simulink model "LUPA_Array_Eqk_circuit_w_PTO_DC_link_v2"  (R2024b)
settings: Solver=VariableStepAuto  StartTime=0.0  StopTime=20  RelTol=1e-5
values from neighbouring files (symbols this model uses):
  B = permute(B,  [3 2 1])    [convh5_v2.m]
  Hs = app.HsField.Value    [WEC_Sankey_App.m]    (also in build_sankey_postprocess.m = output.Hs.x)
  rx = app.DampingField.Value    [WEC_Sankey_App.m]
  sc_factor = 20    [Loss_analysis.m]
  Tp = app.TeField.Value    [WEC_Sankey_App.m]
undefined symbols (not defined in the file or in its folder): C_f1, C_f2, Fex_f1, Fex_f2, hydro, L_hs_f2, lambda, pp, R_cable, R_cable_scaled, R_rad_f1, R_rad_f2, Rs
libraries: fl_lib x41, nesl_utility x24, ee_lib x9
settings Model: Creator=inyongkim  LastModifiedBy=inyongkim
settings DebuggingCC: AlgebraicLoopMsg=none

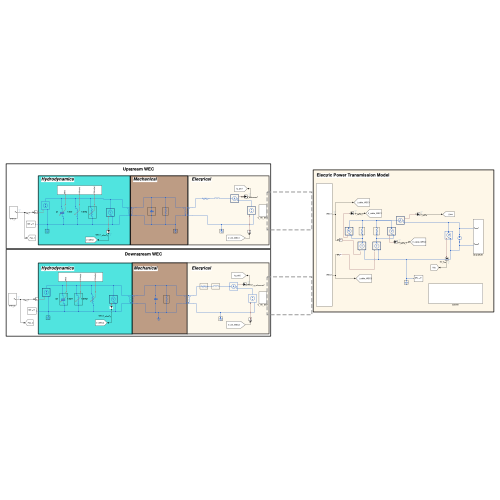
[thumbnail: Simulink's stored preview of the top-level diagram]
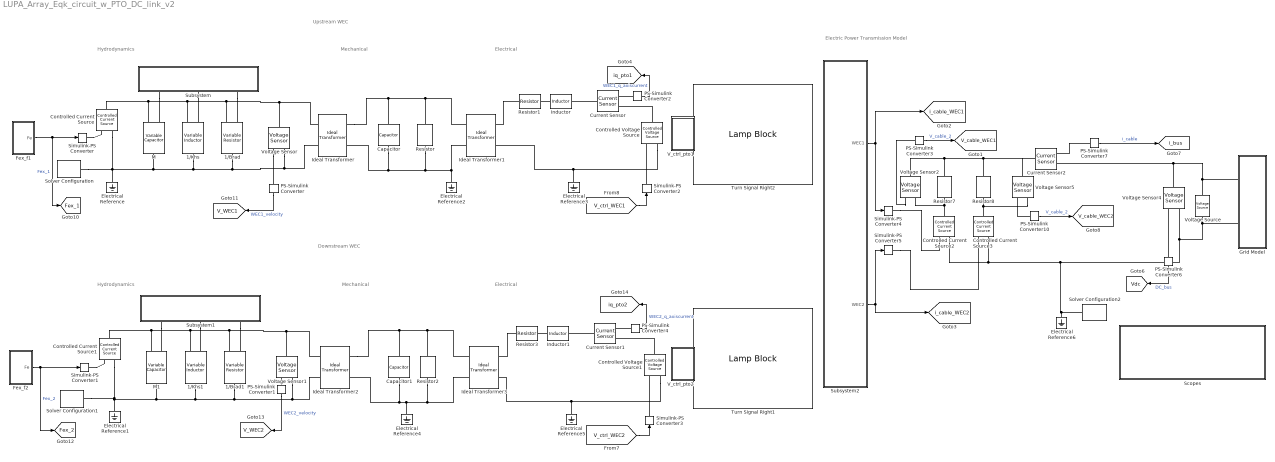
== system LUPA_Array_Eqk_circuit_w_PTO_DC_link_v2 ==
  note: Electrical
  note: Mechanical
  note: Hydrodynamics
  note: Electrical
  note: Mechanical
  note: Hydrodynamics
  note: Electric Power Transmission Model
  note: Upstream WEC
  note: Downstream WEC
  1/Brad : fl_lib/Electrical/Electrical Elements/Variable Resistor  Rmin=0 Ohm  thermalEnable=false  thermal_mass=1 J/K  i_specify=off  i_priority=None  i=0 A  i_nominal_specify=off  i_nominal_value=1  i_nominal_unit=A  v_specify=off  v_priority=None  v=0 V  v_nominal_specify=off  v_nominal_value=1  v_nominal_unit=V  T_specify=off  T_priority=None  T=300 K  T_nominal_specify=off  T_nominal_value=1  T_nominal_unit=K
  1/Brad1 : fl_lib/Electrical/Electrical Elements/Variable Resistor  Rmin=0 Ohm  thermalEnable=false  thermal_mass=1 J/K  i_specify=off  i_priority=None  i=0 A  i_nominal_specify=off  i_nominal_value=1  i_nominal_unit=A  v_specify=off  v_priority=None  v=0 V  v_nominal_specify=off  v_nominal_value=1  v_nominal_unit=V  T_specify=off  T_priority=None  T=300 K  T_nominal_specify=off  T_nominal_value=1  T_nominal_unit=K
  1/Khs : ee_lib/Passive/Variable Inductor  prm=1  Lmin=1e-6 H  g=1e-9 1/Ohm  i0=0 A  phi0=0 Wb
      settings: InternalSimscapePortConfiguration="{\"Bottom\":[],\"Left\":[{\"id\":\"L\",\"label\":\"L\",\"type\":\"input\"},{\"id\":\"p\",\"label\":\"+\",\"type\":\"foundation.electrical.electrical\"}],\"Right\":[{\"id\":\"n\",\"label\":\"-\",\"type\":\"foundation.electrical.electrical\"}],\"Top\":[]}"
  1/Khs1 : ee_lib/Passive/Variable Inductor  prm=1  Lmin=1e-6 H  g=1e-9 1/Ohm  i0=0 A  phi0=0 Wb
      settings: InternalSimscapePortConfiguration="{\"Bottom\":[],\"Left\":[{\"id\":\"L\",\"label\":\"L\",\"type\":\"input\"},{\"id\":\"p\",\"label\":\"+\",\"type\":\"foundation.electrical.electrical\"}],\"Right\":[{\"id\":\"n\",\"label\":\"-\",\"type\":\"foundation.electrical.electrical\"}],\"Top\":[]}"
  Capacitor : fl_lib/Electrical/Electrical Elements/Capacitor  c=J F  r=1e-6 Ohm  g=0 1/Ohm  i_specify=off  i_priority=None  i=0 A  i_nominal_specify=off  i_nominal_value=1  i_nominal_unit=A  v_specify=off  v_priority=None  v=0 V  v_nominal_specify=off  v_nominal_value=1  v_nominal_unit=V  vc_specify=off  vc_priority=High  vc=0 V  vc_nominal_specify=off  vc_nominal_value=1  vc_nominal_unit=V
  Capacitor1 : fl_lib/Electrical/Electrical Elements/Capacitor  c=J F  r=1e-6 Ohm  g=0 1/Ohm  i_specify=off  i_priority=None  i=0 A  i_nominal_specify=off  i_nominal_value=1  i_nominal_unit=A  v_specify=off  v_priority=None  v=0 V  v_nominal_specify=off  v_nominal_value=1  v_nominal_unit=V  vc_specify=off  vc_priority=High  vc=0 V  vc_nominal_specify=off  vc_nominal_value=1  vc_nominal_unit=V
  Controlled Current Source{,1..3} (4 alike) : fl_lib/Electrical/Electrical Sources/Controlled Current Source
  Controlled Voltage Source : fl_lib/Electrical/Electrical Sources/Controlled Voltage Source
  Controlled Voltage Source1 : fl_lib/Electrical/Electrical Sources/Controlled Voltage Source
  Current Sensor : fl_lib/Electrical/Electrical Sensors/Current Sensor
  Current Sensor1 : fl_lib/Electrical/Electrical Sensors/Current Sensor
  Current Sensor2 : fl_lib/Electrical/Electrical Sensors/Current Sensor
  Electrical Reference{,1..6} (7 alike) : fl_lib/Electrical/Electrical Elements/Electrical Reference
  Fex_f1 : Subsystem
  Fex_f2 : Subsystem
  Grid Model : Subsystem
  Ideal Transformer : fl_lib/Electrical/Electrical Elements/Ideal Transformer  n=r  i1_specify=off  i1_priority=None  i1=0 A  i1_nominal_specify=off  i1_nominal_value=1  i1_nominal_unit=A  v1_specify=off  v1_priority=None  v1=0 V  v1_nominal_specify=off  v1_nominal_value=1  v1_nominal_unit=V  i2_specify=off  i2_priority=None  i2=0 A  i2_nominal_specify=off  i2_nominal_value=1  i2_nominal_unit=A  v2_specify=off  v2_priority=None  v2=0 V  v2_nominal_specify=off  v2_nominal_value=1  v2_nominal_unit=V
  Ideal Transformer1 : fl_lib/Electrical/Electrical Elements/Ideal Transformer  n=1/(1.5*lambda*pp)  i1_specify=off  i1_priority=None  i1=0 A  i1_nominal_specify=off  i1_nominal_value=1  i1_nominal_unit=A  v1_specify=off  v1_priority=None  v1=0 V  v1_nominal_specify=off  v1_nominal_value=1  v1_nominal_unit=V  i2_specify=off  i2_priority=None  i2=0 A  i2_nominal_specify=off  i2_nominal_value=1  i2_nominal_unit=A  v2_specify=off  v2_priority=None  v2=0 V  v2_nominal_specify=off  v2_nominal_value=1  v2_nominal_unit=V
  Ideal Transformer2 : fl_lib/Electrical/Electrical Elements/Ideal Transformer  n=r  i1_specify=off  i1_priority=None  i1=0 A  i1_nominal_specify=off  i1_nominal_value=1  i1_nominal_unit=A  v1_specify=off  v1_priority=None  v1=0 V  v1_nominal_specify=off  v1_nominal_value=1  v1_nominal_unit=V  i2_specify=off  i2_priority=None  i2=0 A  i2_nominal_specify=off  i2_nominal_value=1  i2_nominal_unit=A  v2_specify=off  v2_priority=None  v2=0 V  v2_nominal_specify=off  v2_nominal_value=1  v2_nominal_unit=V
  Ideal Transformer3 : fl_lib/Electrical/Electrical Elements/Ideal Transformer  n=1/(1.5*lambda*pp)  i1_specify=off  i1_priority=None  i1=0 A  i1_nominal_specify=off  i1_nominal_value=1  i1_nominal_unit=A  v1_specify=off  v1_priority=None  v1=0 V  v1_nominal_specify=off  v1_nominal_value=1  v1_nominal_unit=V  i2_specify=off  i2_priority=None  i2=0 A  i2_nominal_specify=off  i2_nominal_value=1  i2_nominal_unit=A  v2_specify=off  v2_priority=None  v2=0 V  v2_nominal_specify=off  v2_nominal_value=1  v2_nominal_unit=V
  Inductor : ee_lib/Passive/Inductor  l=Lq H  enable_L_tol=ee.enum.toleranceApplication.none  L_tol=20  tol_distribution=ee.enum.toleranceDistribution.uniform  nSigma=4  r=0 Ohm  g=1e-9 1/Ohm  enable_operating_limits=ee.enum.enable.no  operating_limit_action=ee.enum.passive.reportOpLim.warn  max_working_current=1 A  power_rating=1 W  fault_action=simscape.enum.assert.action.none  t_fault=1 s  i_L_specify=off  i_L_priority=High  i_L=0 A  i_L_nominal_specify=off  i_L_nominal_value=1  i_L_nominal_unit=A
  Inductor1 : ee_lib/Passive/Inductor  l=Lq H  enable_L_tol=ee.enum.toleranceApplication.none  L_tol=20  tol_distribution=ee.enum.toleranceDistribution.uniform  nSigma=4  r=0 Ohm  g=1e-9 1/Ohm  enable_operating_limits=ee.enum.enable.no  operating_limit_action=ee.enum.passive.reportOpLim.warn  max_working_current=1 A  power_rating=1 W  fault_action=simscape.enum.assert.action.none  t_fault=1 s  i_L_specify=off  i_L_priority=High  i_L=0 A  i_L_nominal_specify=off  i_L_nominal_value=1  i_L_nominal_unit=A
  M : ee_lib/Passive/Variable Capacitor  prm=2  Cmin=1e-9 F  r=1e-6 Ohm  v0=0 V  q0=0 C
      settings: InternalSimscapePortConfiguration="{\"Bottom\":[],\"Left\":[{\"id\":\"C\",\"label\":\"C\",\"type\":\"input\"},{\"id\":\"p\",\"label\":\"+\",\"type\":\"foundation.electrical.electrical\"}],\"Right\":[{\"id\":\"n\",\"label\":\"-\",\"type\":\"foundation.electrical.electrical\"}],\"Top\":[]}"
  M1 : ee_lib/Passive/Variable Capacitor  prm=2  Cmin=1e-9 F  r=1e-6 Ohm  v0=0 V  q0=0 C
      settings: InternalSimscapePortConfiguration="{\"Bottom\":[],\"Left\":[{\"id\":\"C\",\"label\":\"C\",\"type\":\"input\"},{\"id\":\"p\",\"label\":\"+\",\"type\":\"foundation.electrical.electrical\"}],\"Right\":[{\"id\":\"n\",\"label\":\"-\",\"type\":\"foundation.electrical.electrical\"}],\"Top\":[]}"
  PS-Simulink Converter{,1..4,6..7,10} (8 alike) : nesl_utility/PS-Simulink Converter  PhysicalDomain=network_engine_domain  SubClassName=ps_output  LeftPortType=input  RightPortType=output  PseudoPeriodic=off  Frequencies=[]  VectorFormat=inherit  Unit=inherit  AffineConversion=off
  Resistor : fl_lib/Electrical/Electrical Elements/Resistor  R=1/B Ohm  i_specify=off  i_priority=None  i=0 A  i_nominal_specify=off  i_nominal_value=1  i_nominal_unit=A  v_specify=off  v_priority=None  v=0 V  v_nominal_specify=off  v_nominal_value=1  v_nominal_unit=V
  Resistor1 : fl_lib/Electrical/Electrical Elements/Resistor  R=Rs Ohm  i_specify=off  i_priority=None  i=0 A  i_nominal_specify=off  i_nominal_value=1  i_nominal_unit=A  v_specify=off  v_priority=None  v=0 V  v_nominal_specify=off  v_nominal_value=1  v_nominal_unit=V
  Resistor2 : fl_lib/Electrical/Electrical Elements/Resistor  R=1/B Ohm  i_specify=off  i_priority=None  i=0 A  i_nominal_specify=off  i_nominal_value=1  i_nominal_unit=A  v_specify=off  v_priority=None  v=0 V  v_nominal_specify=off  v_nominal_value=1  v_nominal_unit=V
  Resistor3 : fl_lib/Electrical/Electrical Elements/Resistor  R=Rs Ohm  i_specify=off  i_priority=None  i=0 A  i_nominal_specify=off  i_nominal_value=1  i_nominal_unit=A  v_specify=off  v_priority=None  v=0 V  v_nominal_specify=off  v_nominal_value=1  v_nominal_unit=V
  Resistor7 : fl_lib/Electrical/Electrical Elements/Resistor  R=R_cable Ohm  i_specify=off  i_priority=None  i=0 A  i_nominal_specify=off  i_nominal_value=1  i_nominal_unit=A  v_specify=off  v_priority=None  v=0 V  v_nominal_specify=off  v_nominal_value=1  v_nominal_unit=V
  Resistor8 : fl_lib/Electrical/Electrical Elements/Resistor  R=R_cable Ohm  i_specify=off  i_priority=None  i=0 A  i_nominal_specify=off  i_nominal_value=1  i_nominal_unit=A  v_specify=off  v_priority=None  v=0 V  v_nominal_specify=off  v_nominal_value=1  v_nominal_unit=V
  Scopes : Subsystem
  Simulink-PS Converter : nesl_utility/Simulink-PS Converter  PhysicalDomain=network_engine_domain  SubClassName=ps_input  LeftPortType=input  RightPortType=output  PseudoPeriodic=off  Frequencies=[]  NoiseDistribution=none  NoiseParameters=[]  Unit=A  AffineConversion=off  FilteringAndDerivatives=provide  SimscapeFilterOrder=1  InputFilterTimeConstant=0.001  UdotUserProvided=0
  Simulink-PS Converter1 : nesl_utility/Simulink-PS Converter  PhysicalDomain=network_engine_domain  SubClassName=ps_input  LeftPortType=input  RightPortType=output  PseudoPeriodic=off  Frequencies=[]  NoiseDistribution=none  NoiseParameters=[]  Unit=A  AffineConversion=off  FilteringAndDerivatives=provide  SimscapeFilterOrder=1  InputFilterTimeConstant=0.001  UdotUserProvided=0
  Simulink-PS Converter{2..5} (4 alike) : nesl_utility/Simulink-PS Converter  PhysicalDomain=network_engine_domain  SubClassName=ps_input  LeftPortType=input  RightPortType=output  PseudoPeriodic=off  Frequencies=[]  NoiseDistribution=none  NoiseParameters=[]  Unit=1  AffineConversion=off  FilteringAndDerivatives=provide  SimscapeFilterOrder=1  InputFilterTimeConstant=0.001  UdotUserProvided=0
  Solver Configuration : nesl_utility/Solver Configuration  PhysicalDomain=network_engine_domain  SubClassName=solver  LeftPortType=input  RightPortType=generic  Tones=[]  Harmonics=[]  SimulateNoise=off  Profile=off  UseLocalSampling=off  EnableSwitchedLinearOptims=on  FrequencyDomain=off  UseCCode=off  RelTol=0.001  AbsTol=0.001  MinStep=1e-09  ToWorkspace=off  RevertToSquareIcSolve=off  NumHomotopyIterations=100  PhasorMode=off  PhasorModeNumHarmonics=1  ConsistencySolver=NEWTON_XTOL_AFTER_FTOL  IndexReductionMethod=DerivativeReplacement  DoDC=off  ResidualTolerance=1e-09  ConsistencyTolSource=GLOBAL  ConsistencyAbsTol=0.001  ConsistencyRelTol=0.001  ConsistencyTolFactor=0.001  UseLocalSolver=off  LocalSolverChoice=NE_BACKWARD_EULER_ADVANCER  ResolveIndetEquations=on  FunctionEvalNumThread=1  LocalSolverSampleTime=0.001  DoFixedCost=off  MaxNonlinIter=3  MaxModeIter=2  ComputeImpulses=off  ImpulseIterations=2  LinearAlgebra=auto  LinearAlgebraNumThread=0  EquationFormulation=NE_TIME_EF  DelaysMemoryBudget=1024  AutomaticFiltering=on  FilteringTimeConstant=0.001  PartitionStorageMethod=AS_NEEDED  PartitionMemoryBudget=1024  PartitionMethod=ROBUST  MultibodyUseLocalSolver=off  MultibodyLocalSolverChoice=ODE1  MultibodyLocalSolverSampleTime=0.001
  Solver Configuration1 : nesl_utility/Solver Configuration  PhysicalDomain=network_engine_domain  SubClassName=solver  LeftPortType=input  RightPortType=generic  Tones=[]  Harmonics=[]  SimulateNoise=off  Profile=off  UseLocalSampling=off  EnableSwitchedLinearOptims=on  FrequencyDomain=off  UseCCode=off  RelTol=0.001  AbsTol=0.001  MinStep=1e-09  ToWorkspace=off  RevertToSquareIcSolve=off  NumHomotopyIterations=100  PhasorMode=off  PhasorModeNumHarmonics=1  ConsistencySolver=NEWTON_XTOL_AFTER_FTOL  IndexReductionMethod=DerivativeReplacement  DoDC=off  ResidualTolerance=1e-09  ConsistencyTolSource=GLOBAL  ConsistencyAbsTol=0.001  ConsistencyRelTol=0.001  ConsistencyTolFactor=0.001  UseLocalSolver=off  LocalSolverChoice=NE_BACKWARD_EULER_ADVANCER  ResolveIndetEquations=on  FunctionEvalNumThread=1  LocalSolverSampleTime=0.001  DoFixedCost=off  MaxNonlinIter=3  MaxModeIter=2  ComputeImpulses=off  ImpulseIterations=2  LinearAlgebra=auto  LinearAlgebraNumThread=0  EquationFormulation=NE_TIME_EF  DelaysMemoryBudget=1024  AutomaticFiltering=on  FilteringTimeConstant=0.001  PartitionStorageMethod=AS_NEEDED  PartitionMemoryBudget=1024  PartitionMethod=ROBUST  MultibodyUseLocalSolver=off  MultibodyLocalSolverChoice=ODE1  MultibodyLocalSolverSampleTime=0.001
  Solver Configuration2 : nesl_utility/Solver Configuration  PhysicalDomain=network_engine_domain  SubClassName=solver  LeftPortType=input  RightPortType=generic  Tones=[]  Harmonics=[]  SimulateNoise=off  Profile=off  UseLocalSampling=off  EnableSwitchedLinearOptims=on  FrequencyDomain=off  UseCCode=off  RelTol=0.001  AbsTol=0.001  MinStep=1e-09  ToWorkspace=off  RevertToSquareIcSolve=off  NumHomotopyIterations=100  PhasorMode=off  PhasorModeNumHarmonics=1  ConsistencySolver=NEWTON_XTOL_AFTER_FTOL  IndexReductionMethod=DerivativeReplacement  DoDC=off  ResidualTolerance=1e-09  ConsistencyTolSource=GLOBAL  ConsistencyAbsTol=0.001  ConsistencyRelTol=0.001  ConsistencyTolFactor=0.001  UseLocalSolver=off  LocalSolverChoice=NE_BACKWARD_EULER_ADVANCER  ResolveIndetEquations=on  FunctionEvalNumThread=1  LocalSolverSampleTime=0.001  DoFixedCost=off  MaxNonlinIter=3  MaxModeIter=2  ComputeImpulses=off  ImpulseIterations=2  LinearAlgebra=auto  LinearAlgebraNumThread=0  EquationFormulation=NE_TIME_EF  DelaysMemoryBudget=1024  AutomaticFiltering=on  FilteringTimeConstant=0.001  PartitionStorageMethod=AS_NEEDED  PartitionMemoryBudget=1024  PartitionMethod=ROBUST  MultibodyUseLocalSolver=off  MultibodyLocalSolverChoice=ODE1  MultibodyLocalSolverSampleTime=0.001
  Subsystem : Subsystem
  Subsystem1 : Subsystem
  Subsystem2 : Subsystem
  Turn Signal Right1 : LampBlock  LabelPosition=Hide  Icon=TurnSignalRight
  Turn Signal Right2 : LampBlock  LabelPosition=Hide  Icon=TurnSignalRight
  V_ctrl_pto1 : Subsystem
  V_ctrl_pto2 : Subsystem
  Voltage Sensor{,1..2,4..5} (5 alike) : fl_lib/Electrical/Electrical Sensors/Voltage Sensor
  Voltage Source : ee_lib/Sources/Voltage Source  dc_voltage=V_grid_scaled V  ac_voltage=0 V  ac_shift=0 rad  ac_frequency=60 Hz  noise_mode=ee.enum.sources.noise.Disabled  PSD=0 V^2/Hz  sample_time=1e-3 s  repeatability=ee.enum.sources.repeatability.NotRepeatable  user_seed=0  auto_seed=3499211588  i_specify=off  i_priority=None  i=0 A  i_nominal_specify=off  i_nominal_value=1  i_nominal_unit=A  v_specify=off  v_priority=None  v=0 V  v_nominal_specify=off  v_nominal_value=1  v_nominal_unit=V
  tag scope: Fex_1=global, Fex_2=global, V_WEC1=global, V_WEC2=global, V_cable_WEC1=global, V_cable_WEC2=global, Vdc=global, i_bus=global, i_cable_WEC1=global, i_cable_WEC2=global, iq_pto1=global, iq_pto2=global
  wires:
  Fex_f2/1(Fe) -> [Fex_2], Simulink-PS Converter1/1  "Fex_2"
  PS-Simulink Converter/1 -> [V_WEC1]  "WEC1_velocity"
  Subsystem2/1(WEC1) -> [i_cable_WEC1], Simulink-PS Converter4/1
  [V_ctrl_WEC1] -> Simulink-PS Converter2/1
  PS-Simulink Converter10/1 -> [V_cable_WEC2]  "V_cable_2"
  PS-Simulink Converter6/1 -> [Vdc]  "DC_bus"
  PS-Simulink Converter3/1 -> [V_cable_WEC1]  "V_cable_2"
  Fex_f1/1(Fe) -> [Fex_1], Simulink-PS Converter/1  "Fex_1"
  PS-Simulink Converter7/1 -> [i_bus]  "i_cable"
  PS-Simulink Converter4/1 -> [iq_pto2]  "WEC2_q_axiscurrent"
  PS-Simulink Converter1/1 -> [V_WEC2]  "WEC2_velocity"
  PS-Simulink Converter2/1 -> [iq_pto1]  "WEC1_q_axiscurrent"
  Subsystem2/2(WEC2) -> Simulink-PS Converter5/1, [i_cable_WEC2]
  [V_ctrl_WEC2] -> Simulink-PS Converter3/1
  connections:
  Resistor3/LConn1 -- Ideal Transformer3/RConn1
  Current Sensor/LConn1 -- Inductor/RConn1
  PS-Simulink Converter10/LConn1 -- Voltage Sensor5/RConn1
  Resistor8/LConn1 -- Voltage Sensor5/RConn2 -- Controlled Current Source3/LConn1
  Current Sensor1/LConn1 -- Inductor1/RConn1
  M1/RConn1 -- Controlled Current Source1/RConn2 -- Solver Configuration1/RConn1 -- Electrical Reference1/LConn1 -- Ideal Transformer2/LConn2 -- Voltage Sensor1/RConn2 -- 1/Brad1/RConn1 -- 1/Khs1/RConn1
  Inductor/LConn1 -- Resistor1/RConn1
  Ideal Transformer2/RConn1 -- Ideal Transformer3/LConn1 -- Resistor2/LConn1 -- Capacitor1/LConn1
  Subsystem1/RConn2 -- 1/Khs1/LConn1
  Controlled Voltage Source1/RConn2 -- Electrical Reference5/LConn1 -- Ideal Transformer3/RConn2
  Controlled Current Source/RConn2 -- Solver Configuration/RConn1 -- Electrical Reference/LConn1 -- Ideal Transformer/LConn2 -- Voltage Sensor/RConn2 -- 1/Brad/RConn1 -- 1/Khs/RConn1 -- M/RConn1
  Simulink-PS Converter5/RConn1 -- Controlled Current Source3/RConn1
  Current Sensor2/RConn2 -- Voltage Sensor4/LConn1 -- Voltage Source/LConn1 -- Grid Model/LConn1
  PS-Simulink Converter4/LConn1 -- Current Sensor1/RConn1
  Ideal Transformer3/LConn2 -- Resistor2/RConn1 -- Capacitor1/RConn1 -- Ideal Transformer2/RConn2 -- Electrical Reference4/LConn1
  Subsystem1/RConn1 -- M1/LConn1
  Voltage Sensor1/RConn1 -- PS-Simulink Converter1/LConn1
  Controlled Voltage Source1/LConn1 -- Current Sensor1/RConn2
  Subsystem1/RConn3 -- 1/Brad1/LConn1
  Capacitor/RConn1 -- Electrical Reference2/LConn1 -- Ideal Transformer1/LConn2 -- Resistor/RConn1 -- Ideal Transformer/RConn2
  Controlled Current Source/LConn1 -- Voltage Sensor/LConn1 -- Ideal Transformer/LConn1 -- 1/Brad/LConn2 -- 1/Khs/LConn2 -- M/LConn2
  Simulink-PS Converter3/RConn1 -- Controlled Voltage Source1/RConn1
  Resistor1/LConn1 -- Ideal Transformer1/RConn1
  Ideal Transformer/RConn1 -- Ideal Transformer1/LConn1 -- Resistor/LConn1 -- Capacitor/LConn1
  PS-Simulink Converter2/LConn1 -- Current Sensor/RConn1
  Subsystem/RConn3 -- 1/Brad/LConn1
  Subsystem/RConn2 -- 1/Khs/LConn1
  Simulink-PS Converter1/RConn1 -- Controlled Current Source1/RConn1
  Controlled Current Source2/LConn1 -- Voltage Sensor2/RConn2 -- Resistor7/LConn1
  Simulink-PS Converter2/RConn1 -- Controlled Voltage Source/RConn1
  1/Khs1/LConn2 -- Controlled Current Source1/LConn1 -- M1/LConn2 -- Voltage Sensor1/LConn1 -- Ideal Transformer2/LConn1 -- 1/Brad1/LConn2
  PS-Simulink Converter7/LConn1 -- Current Sensor2/RConn1
  Solver Configuration2/RConn1 -- Controlled Current Source3/RConn2 -- Controlled Current Source2/RConn2 -- Voltage Source/RConn1 -- Grid Model/LConn2 -- Voltage Sensor4/RConn2 -- Electrical Reference6/LConn1
  PS-Simulink Converter6/LConn1 -- Voltage Sensor4/RConn1
  Simulink-PS Converter/RConn1 -- Controlled Current Source/RConn1
  Voltage Sensor/RConn1 -- PS-Simulink Converter/LConn1
  Resistor7/RConn1 -- Voltage Sensor2/LConn1 -- Voltage Sensor5/LConn1 -- Current Sensor2/LConn1 -- Resistor8/RConn1
  Controlled Voltage Source/LConn1 -- Current Sensor/RConn2
  Subsystem/RConn1 -- M/LConn1
  Inductor1/LConn1 -- Resistor3/RConn1
  Simulink-PS Converter4/RConn1 -- Controlled Current Source2/RConn1
  Controlled Voltage Source/RConn2 -- Electrical Reference3/LConn1 -- Ideal Transformer1/RConn2
  Voltage Sensor2/RConn1 -- PS-Simulink Converter3/LConn1

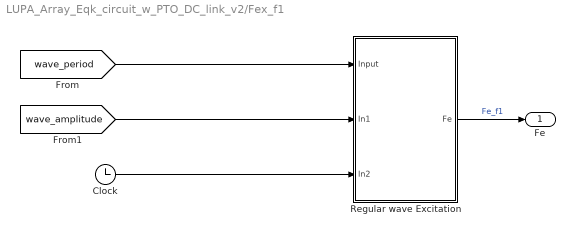
== system LUPA_Array_Eqk_circuit_w_PTO_DC_link_v2/Fex_f1 ==
  Clock : Clock
  Regular wave Excitation : Subsystem
  Fe : Outport
  wires:
  Regular wave Excitation/1(Fe) -> Fe/1  "Fe_f1"
  Clock/1 -> Regular wave Excitation/3(In2)
  [wave_period] -> Regular wave Excitation/1(Input)
  [wave_amplitude] -> Regular wave Excitation/2(In1)

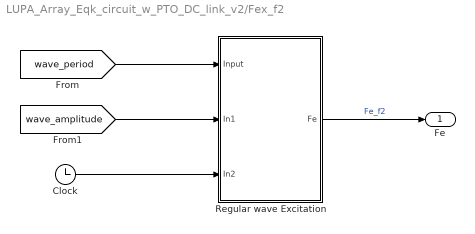
== system LUPA_Array_Eqk_circuit_w_PTO_DC_link_v2/Fex_f2 ==
  Clock : Clock
  Regular wave Excitation : Subsystem
  Fe : Outport
  wires:
  Regular wave Excitation/1(Fe) -> Fe/1  "Fe_f2"
  Clock/1 -> Regular wave Excitation/3(In2)
  [wave_amplitude] -> Regular wave Excitation/2(In1)
  [wave_period] -> Regular wave Excitation/1(Input)

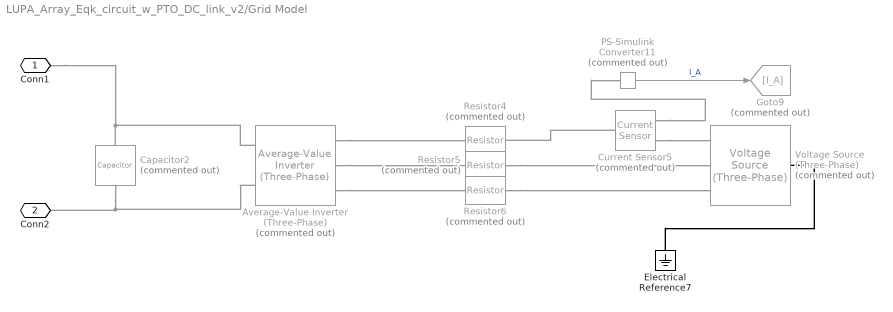
== system LUPA_Array_Eqk_circuit_w_PTO_DC_link_v2/Grid Model ==
  Average-Value Inverter (Three-Phase) : ee_lib/Semiconductors & Converters/Converters/Average-Value Inverter (Three-Phase)  Commented=on  port_option=ee.enum.threePhasePort.expanded  FRated=f_scaled Hz  PhaseShift=0 deg  voltage_ratio=sqrt(6) / pi  Pfixed=1e3*sc_factor^3.5 W  v_on=100*sc_factor^1.25 V  v_off=75*sc_factor^1.25 V
      settings: InternalSimscapePortConfiguration="{\"Bottom\":[],\"Left\":[{\"id\":\"p\",\"label\":\"+\",\"type\":\"foundation.electrical.electrical\"},{\"id\":\"n\",\"label\":\"-\",\"type\":\"foundation.electrical.electrical\"}],\"Right\":[{\"id\":\"a\",\"label\":\"a\",\"type\":\"foundation.electrical.electrical\"},{\"id\":\"b\",\"label\":\"b\",\"type\":\"foundation.electrical.electrical\"},{\"id\":\"c\",\"label\":\"c\",\"type\":\"foundation.electrical.electrical\"}],\"Top\":[]}"
  Capacitor2 : fl_lib/Electrical/Electrical Elements/Capacitor  Commented=on  c=1e-6 F  r=1e-6 Ohm  g=0 1/Ohm  i_specify=off  i_priority=None  i=0 A  i_nominal_specify=off  i_nominal_value=1  i_nominal_unit=A  v_specify=on  v_priority=None  v=300 V  v_nominal_specify=off  v_nominal_value=1  v_nominal_unit=V  vc_specify=off  vc_priority=High  vc=0 V  vc_nominal_specify=off  vc_nominal_value=1  vc_nominal_unit=V
  Current Sensor5 : fl_lib/Electrical/Electrical Sensors/Current Sensor  Commented=on
  Electrical Reference7 : fl_lib/Electrical/Electrical Elements/Electrical Reference
  Goto9 : Goto  Commented=on  GotoTag=I_A
  PS-Simulink Converter11 : nesl_utility/PS-Simulink Converter  Commented=on  PhysicalDomain=network_engine_domain  SubClassName=ps_output  LeftPortType=input  RightPortType=output  PseudoPeriodic=off  Frequencies=[]  VectorFormat=inherit  Unit=inherit  AffineConversion=off
  Resistor4 : fl_lib/Electrical/Electrical Elements/Resistor  Commented=on  R=R_cable_scaled Ohm  i_specify=off  i_priority=None  i=0 A  i_nominal_specify=off  i_nominal_value=1  i_nominal_unit=A  v_specify=off  v_priority=None  v=0 V  v_nominal_specify=off  v_nominal_value=1  v_nominal_unit=V
  Resistor5 : fl_lib/Electrical/Electrical Elements/Resistor  Commented=on  R=R_cable_scaled Ohm  i_specify=off  i_priority=None  i=0 A  i_nominal_specify=off  i_nominal_value=1  i_nominal_unit=A  v_specify=off  v_priority=None  v=0 V  v_nominal_specify=off  v_nominal_value=1  v_nominal_unit=V
  Resistor6 : fl_lib/Electrical/Electrical Elements/Resistor  Commented=on  R=R_cable_scaled Ohm  i_specify=off  i_priority=None  i=0 A  i_nominal_specify=off  i_nominal_value=1  i_nominal_unit=A  v_specify=off  v_priority=None  v=0 V  v_nominal_specify=off  v_nominal_value=1  v_nominal_unit=V
  Voltage Source (Three-Phase) : ee_lib/Sources/Voltage Source (Three-Phase)  Commented=on  vline_rms=V_grid_scaled_AC V  shift=0 deg  freq=f_scaled Hz  impedance_option=1  SShortCircuit=1e6*sc_factor^3.5 A*V  XR=15  R=0.01 Ohm  L=3.97e-4 H  harmonic_option=0  harmonic_orders=[5, 7, 11, 13]  harmonic_ratios=[.1, .1, .1, .1]  G_parasitic=0 1/Ohm  I_specify=off  I_priority=None  I=[0, 0, 0] A  I_nominal_specify=off  I_nominal_value=1  I_nominal_unit=A
      settings: InternalSimscapePortConfiguration="{\"Bottom\":[],\"Left\":[{\"id\":\"n\",\"label\":\"n\",\"type\":\"foundation.electrical.electrical\"}],\"Right\":[{\"id\":\"a\",\"label\":\"a\",\"type\":\"foundation.electrical.electrical\"},{\"id\":\"b\",\"label\":\"b\",\"type\":\"foundation.electrical.electrical\"},{\"id\":\"c\",\"label\":\"c\",\"type\":\"foundation.electrical.electrical\"}],\"Top\":[]}"
  Conn1 : PMIOPort  Side=Left
  Conn2 : PMIOPort  Port=2  Side=Left
  wires:
  PS-Simulink Converter11/1 -> Goto9/1  "I_A"
  connections:
  Resistor6/RConn1 -- Voltage Source (Three-Phase)/RConn1
  Current Sensor5/RConn2 -- Voltage Source (Three-Phase)/RConn3
  Average-Value Inverter (Three-Phase)/RConn2 -- Resistor5/LConn1
  Average-Value Inverter (Three-Phase)/RConn3 -- Resistor6/LConn1
  Average-Value Inverter (Three-Phase)/LConn2 -- Conn2/RConn1 -- Capacitor2/RConn1
  Current Sensor5/LConn1 -- Resistor4/RConn1
  Average-Value Inverter (Three-Phase)/RConn1 -- Resistor4/LConn1
  Current Sensor5/RConn1 -- PS-Simulink Converter11/LConn1
  Electrical Reference7/LConn1 -- Voltage Source (Three-Phase)/LConn1
  Capacitor2/LConn1 -- Conn1/RConn1 -- Average-Value Inverter (Three-Phase)/LConn1
  Resistor5/RConn1 -- Voltage Source (Three-Phase)/RConn2

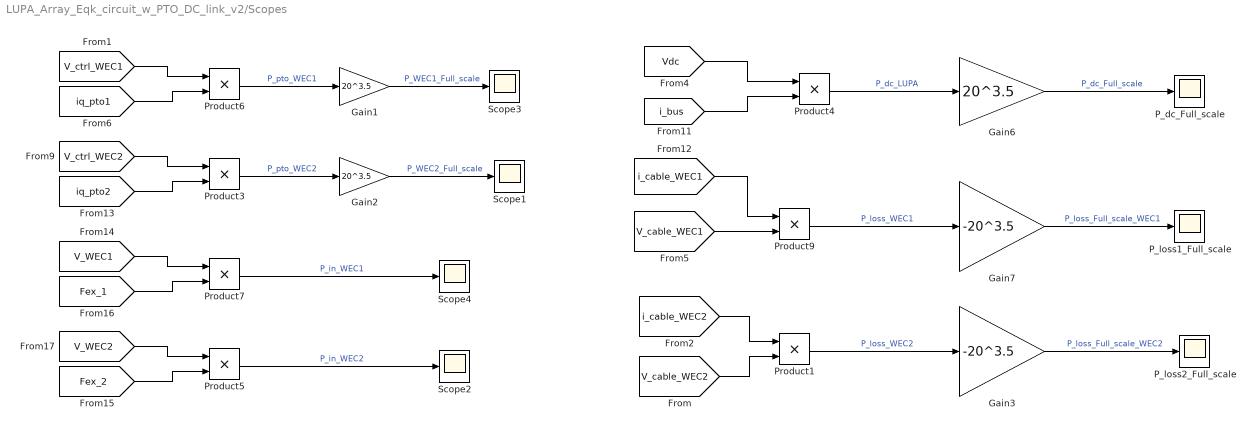
== system LUPA_Array_Eqk_circuit_w_PTO_DC_link_v2/Scopes ==
  Gain1 : Gain  Gain=20^3.5
  Gain2 : Gain  Gain=20^3.5
  Gain3 : Gain  Gain=-20^3.5
  Gain6 : Gain  Gain=20^3.5
  Gain7 : Gain  Gain=-20^3.5
  P_dc_Full_scale : Scope
  P_loss1_Full_scale : Scope
  P_loss2_Full_scale : Scope
  Product{1,3..7,9} (7 alike) : Product
  Scope{1..4} (4 alike) : Scope
  wires:
  [iq_pto1] -> Product6/2
  [i_bus] -> Product4/2
  [i_cable_WEC1] -> Product9/1
  [V_WEC2] -> Product5/1
  [Fex_2] -> Product5/2
  [Fex_1] -> Product7/2
  [V_ctrl_WEC1] -> Product6/1
  Gain1/1 -> Scope3/1  "P_WEC1_Full_scale"
  [V_WEC1] -> Product7/1
  Product7/1 -> Scope4/1  "P_in_WEC1"
  Product5/1 -> Scope2/1  "P_in_WEC2"
  Product3/1 -> Gain2/1  "P_pto_WEC2"
  Product6/1 -> Gain1/1  "P_pto_WEC1"
  Gain7/1 -> P_loss1_Full_scale/1  "P_loss_Full_scale_WEC1"
  [V_ctrl_WEC2] -> Product3/1
  [iq_pto2] -> Product3/2
  [V_cable_WEC1] -> Product9/2
  Gain6/1 -> P_dc_Full_scale/1  "P_dc_Full_scale"
  [Vdc] -> Product4/1
  Product4/1 -> Gain6/1  "P_dc_LUPA"
  Product9/1 -> Gain7/1  "P_loss_WEC1"
  Gain2/1 -> Scope1/1  "P_WEC2_Full_scale"
  [i_cable_WEC2] -> Product1/1
  [V_cable_WEC2] -> Product1/2
  Product1/1 -> Gain3/1  "P_loss_WEC2"
  Gain3/1 -> P_loss2_Full_scale/1  "P_loss_Full_scale_WEC2"

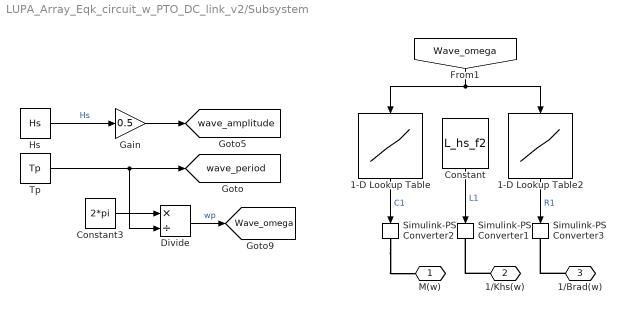
== system LUPA_Array_Eqk_circuit_w_PTO_DC_link_v2/Subsystem ==
  1-D Lookup Table : Lookup_n-D  NumberOfTableDimensions=1  BreakpointsForDimension1=hydro.w  Table=C_f1  InternalRulePriority=Speed  RndMeth=Simplest
  1-D Lookup Table2 : Lookup_n-D  NumberOfTableDimensions=1  BreakpointsForDimension1=hydro.w  Table=R_rad_f1  InternalRulePriority=Speed  RndMeth=Simplest
  Constant : Constant  Value=L_hs_f2
  Constant3 : Constant  Value=2*pi
  Divide : Product  Inputs=*/
  Gain : Gain  Gain=0.5
  Hs : Constant  Value=Hs
  Simulink-PS Converter1 : nesl_utility/Simulink-PS Converter  PhysicalDomain=network_engine_domain  SubClassName=ps_input  LeftPortType=input  RightPortType=output  PseudoPeriodic=off  Frequencies=[]  NoiseDistribution=none  NoiseParameters=[]  Unit=1  AffineConversion=off  FilteringAndDerivatives=provide  SimscapeFilterOrder=1  InputFilterTimeConstant=0.001  UdotUserProvided=0
  Simulink-PS Converter2 : nesl_utility/Simulink-PS Converter  PhysicalDomain=network_engine_domain  SubClassName=ps_input  LeftPortType=input  RightPortType=output  PseudoPeriodic=off  Frequencies=[]  NoiseDistribution=none  NoiseParameters=[]  Unit=1  AffineConversion=off  FilteringAndDerivatives=provide  SimscapeFilterOrder=1  InputFilterTimeConstant=0.001  UdotUserProvided=0
  Simulink-PS Converter3 : nesl_utility/Simulink-PS Converter  PhysicalDomain=network_engine_domain  SubClassName=ps_input  LeftPortType=input  RightPortType=output  PseudoPeriodic=off  Frequencies=[]  NoiseDistribution=none  NoiseParameters=[]  Unit=1  AffineConversion=off  FilteringAndDerivatives=provide  SimscapeFilterOrder=1  InputFilterTimeConstant=0.001  UdotUserProvided=0
  Tp : Constant  Value=Tp
  M(w) : PMIOPort  Side=Right
  1/Khs(w) : PMIOPort  Port=2  Side=Right
  1/Brad(w) : PMIOPort  Port=3  Side=Right
  tag scope: Wave_omega=global, wave_amplitude=global, wave_period=global
  wires:
  1-D Lookup Table/1 -> Simulink-PS Converter2/1  "C1"
  [Wave_omega] -> 1-D Lookup Table2/1, 1-D Lookup Table/1
  1-D Lookup Table2/1 -> Simulink-PS Converter3/1  "R1"
  Constant/1 -> Simulink-PS Converter1/1  "L1"
  Hs/1 -> Gain/1  "Hs"
  Constant3/1 -> Divide/1
  Tp/1 -> Divide/2, [wave_period]
  Gain/1 -> [wave_amplitude]
  Divide/1 -> [Wave_omega]  "wp"
  connections:
  1/Brad(w)/RConn1 -- Simulink-PS Converter3/RConn1
  1/Khs(w)/RConn1 -- Simulink-PS Converter1/RConn1
  Simulink-PS Converter2/RConn1 -- M(w)/RConn1

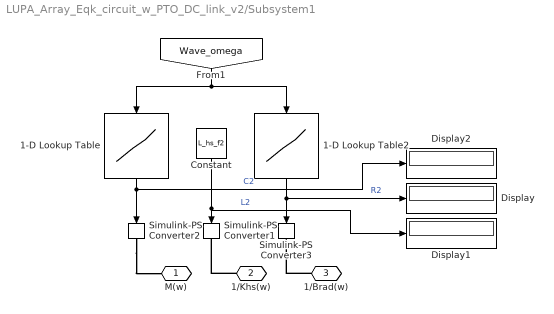
== system LUPA_Array_Eqk_circuit_w_PTO_DC_link_v2/Subsystem1 ==
  1-D Lookup Table : Lookup_n-D  NumberOfTableDimensions=1  BreakpointsForDimension1=hydro.w  Table=C_f2  InternalRulePriority=Speed  RndMeth=Simplest
  1-D Lookup Table2 : Lookup_n-D  NumberOfTableDimensions=1  BreakpointsForDimension1=hydro.w  Table=R_rad_f2  InternalRulePriority=Speed  RndMeth=Simplest
  Constant : Constant  Value=L_hs_f2
  Display : Display
  Display1 : Display
  Display2 : Display
  Simulink-PS Converter1 : nesl_utility/Simulink-PS Converter  PhysicalDomain=network_engine_domain  SubClassName=ps_input  LeftPortType=input  RightPortType=output  PseudoPeriodic=off  Frequencies=[]  NoiseDistribution=none  NoiseParameters=[]  Unit=1  AffineConversion=off  FilteringAndDerivatives=provide  SimscapeFilterOrder=1  InputFilterTimeConstant=0.001  UdotUserProvided=0
  Simulink-PS Converter2 : nesl_utility/Simulink-PS Converter  PhysicalDomain=network_engine_domain  SubClassName=ps_input  LeftPortType=input  RightPortType=output  PseudoPeriodic=off  Frequencies=[]  NoiseDistribution=none  NoiseParameters=[]  Unit=1  AffineConversion=off  FilteringAndDerivatives=provide  SimscapeFilterOrder=1  InputFilterTimeConstant=0.001  UdotUserProvided=0
  Simulink-PS Converter3 : nesl_utility/Simulink-PS Converter  PhysicalDomain=network_engine_domain  SubClassName=ps_input  LeftPortType=input  RightPortType=output  PseudoPeriodic=off  Frequencies=[]  NoiseDistribution=none  NoiseParameters=[]  Unit=1  AffineConversion=off  FilteringAndDerivatives=provide  SimscapeFilterOrder=1  InputFilterTimeConstant=0.001  UdotUserProvided=0
  M(w) : PMIOPort  Side=Right
  1/Khs(w) : PMIOPort  Port=2  Side=Right
  1/Brad(w) : PMIOPort  Port=3  Side=Right
  wires:
  [Wave_omega] -> 1-D Lookup Table2/1, 1-D Lookup Table/1
  1-D Lookup Table/1 -> Simulink-PS Converter2/1, Display2/1  "C2"
  Constant/1 -> Display1/1, Simulink-PS Converter1/1  "L2"
  1-D Lookup Table2/1 -> Display/1, Simulink-PS Converter3/1  "R2"
  connections:
  1/Brad(w)/RConn1 -- Simulink-PS Converter3/RConn1
  1/Khs(w)/RConn1 -- Simulink-PS Converter1/RConn1
  Simulink-PS Converter2/RConn1 -- M(w)/RConn1

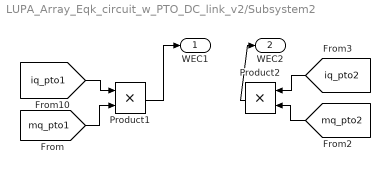
== system LUPA_Array_Eqk_circuit_w_PTO_DC_link_v2/Subsystem2 ==
  Product1 : Product
  Product2 : Product
  WEC1 : Outport
  WEC2 : Outport  Port=2
  wires:
  [iq_pto2] -> Product2/1
  Product2/1 -> WEC2/1
  Product1/1 -> WEC1/1
  [mq_pto2] -> Product2/2
  [mq_pto1] -> Product1/2
  [iq_pto1] -> Product1/1

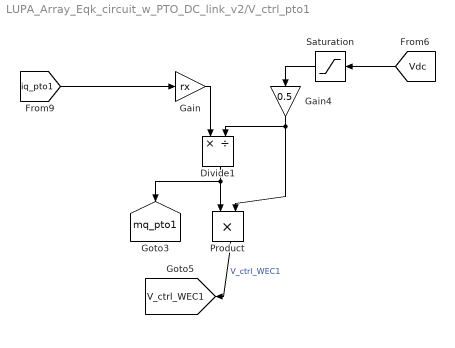
== system LUPA_Array_Eqk_circuit_w_PTO_DC_link_v2/V_ctrl_pto1 ==
  Divide1 : Product  Inputs=*/
  Gain : Gain  Gain=rx
  Gain4 : Gain  Gain=0.5
  Product : Product
  Saturation : Saturate  UpperLimit=1000  LowerLimit=-1000
  tag scope: V_ctrl_WEC1=global, mq_pto1=global
  wires:
  [Vdc] -> Saturation/1
  Divide1/1 -> [mq_pto1], Product/1
  [iq_pto1] -> Gain/1
  Product/1 -> [V_ctrl_WEC1]  "V_ctrl_WEC1"
  Gain/1 -> Divide1/1
  Saturation/1 -> Gain4/1
  Gain4/1 -> Product/2, Divide1/2

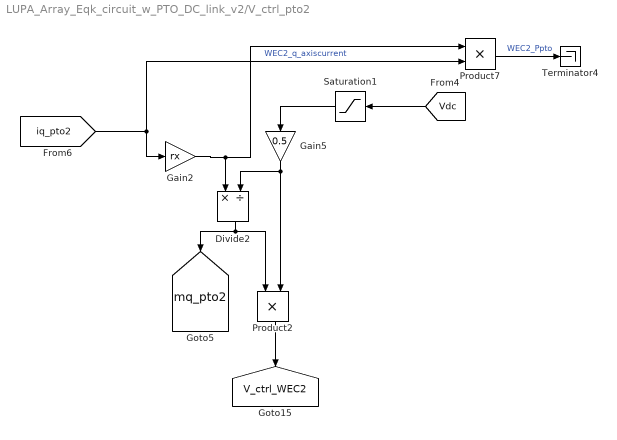
== system LUPA_Array_Eqk_circuit_w_PTO_DC_link_v2/V_ctrl_pto2 ==
  Divide2 : Product  Inputs=*/
  Gain2 : Gain  Gain=rx
  Gain5 : Gain  Gain=0.5
  Product2 : Product
  Product7 : Product
  Saturation1 : Saturate  UpperLimit=1000  LowerLimit=-1000
  Terminator4 : Terminator
  tag scope: V_ctrl_WEC2=global, mq_pto2=global
  wires:
  [Vdc] -> Saturation1/1
  Divide2/1 -> [mq_pto2], Product2/1
  Gain5/1 -> Product2/2, Divide2/2
  Product7/1 -> Terminator4/1  "WEC2_Ppto"
  [iq_pto2] -> Gain2/1, Product7/2  "WEC2_q_axiscurrent"
  Product2/1 -> [V_ctrl_WEC2]
  Saturation1/1 -> Gain5/1
  Gain2/1 -> Product7/1, Divide2/1

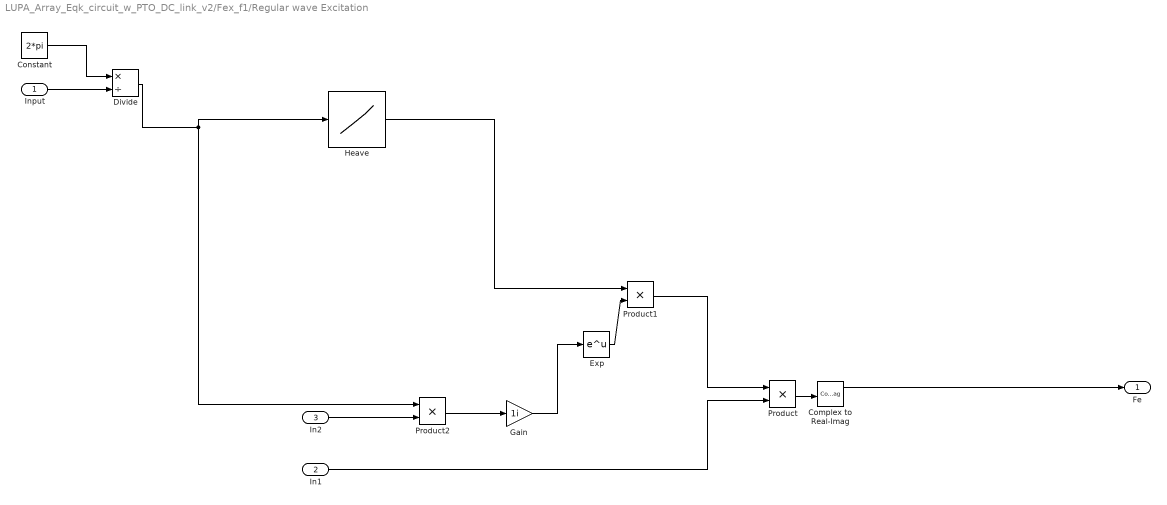
== system LUPA_Array_Eqk_circuit_w_PTO_DC_link_v2/Fex_f1/Regular wave Excitation ==
  Input : Inport
  In1 : Inport  Port=2
  In2 : Inport  Port=3
  Complex to Real-Imag : ComplexToRealImag
  Constant : Constant  Value=2*pi
  Divide : Product  Inputs=*/
  Exp : Math
  Gain : Gain  Gain=1i
  Heave : Lookup_n-D  NumberOfTableDimensions=1  BreakpointsForDimension1=hydro.w  Table=Fex_f1(3,:)  InternalRulePriority=Speed  RndMeth=Simplest
  Product : Product
  Product1 : Product
  Product2 : Product
  Fe : Outport
  wires:
  Complex to Real-Imag/1 -> Fe/1
  Divide/1 -> Heave/1, Product2/1
  Product1/1 -> Product/1
  In1/1 -> Product/2
  In2/1 -> Product2/2
  Product2/1 -> Gain/1
  Gain/1 -> Exp/1
  Exp/1 -> Product1/2
  Product/1 -> Complex to Real-Imag/1
  Heave/1 -> Product1/1
  Input/1 -> Divide/2
  Constant/1 -> Divide/1

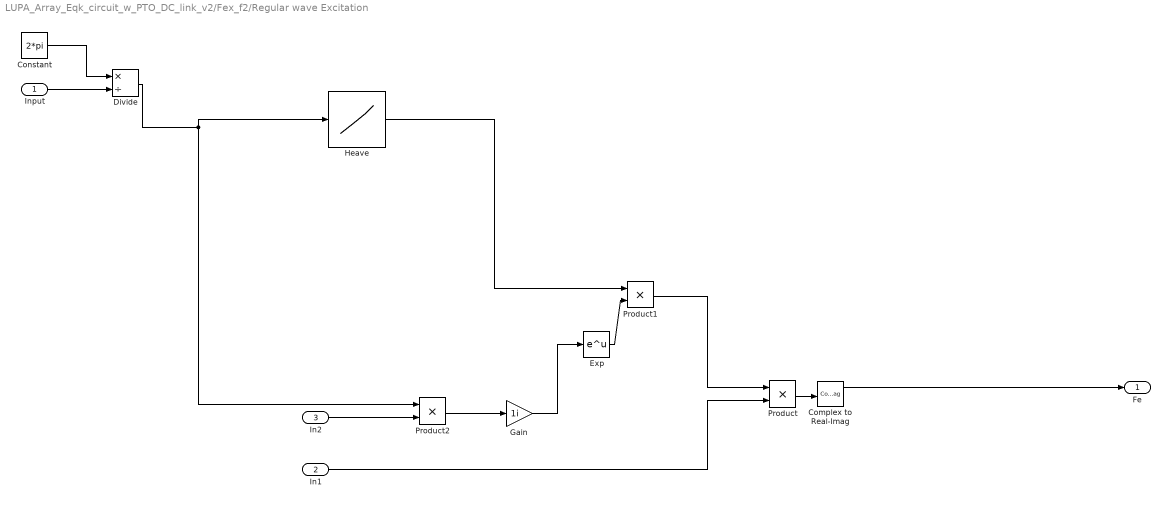
== system LUPA_Array_Eqk_circuit_w_PTO_DC_link_v2/Fex_f2/Regular wave Excitation ==
  Input : Inport
  In1 : Inport  Port=2
  In2 : Inport  Port=3
  Complex to Real-Imag : ComplexToRealImag
  Constant : Constant  Value=2*pi
  Divide : Product  Inputs=*/
  Exp : Math
  Gain : Gain  Gain=1i
  Heave : Lookup_n-D  NumberOfTableDimensions=1  BreakpointsForDimension1=hydro.w  Table=Fex_f2(3,:)  InternalRulePriority=Speed  RndMeth=Simplest
  Product : Product
  Product1 : Product
  Product2 : Product
  Fe : Outport
  wires:
  Complex to Real-Imag/1 -> Fe/1
  Divide/1 -> Heave/1, Product2/1
  Product1/1 -> Product/1
  In1/1 -> Product/2
  In2/1 -> Product2/2
  Product2/1 -> Gain/1
  Gain/1 -> Exp/1
  Exp/1 -> Product1/2
  Product/1 -> Complex to Real-Imag/1
  Heave/1 -> Product1/1
  Input/1 -> Divide/2
  Constant/1 -> Divide/1
